simulink model "SimpleBounce"  (Simulink 10.0)
settings: Solver=ode23t  StartTime=0.0  StopTime=3  RelTol=1e-3  EnableMultiTasking=on
libraries: simulink x1, tstbxlib x1
settings Model: Creator=grouleau  LastModifiedBy=bhisma
settings SolverCC: ZeroCrossControl=EnableAll
settings DataIOCC: LimitDataPoints=on  SignalLoggingSaveFormat=ModelDataLogs
settings OptimizationCC: ExpressionDepthLimit=2147483647
settings DebuggingCC: SolverPrmCheckMsg=warning  FcnCallInpInsideContextMsg=warning  StateNameClashWarn=warning
settings GRTTargetCC: GeneratePreprocessorConditionals=Disable all
settings ConfigComp: CovExternalEMLEnable=off

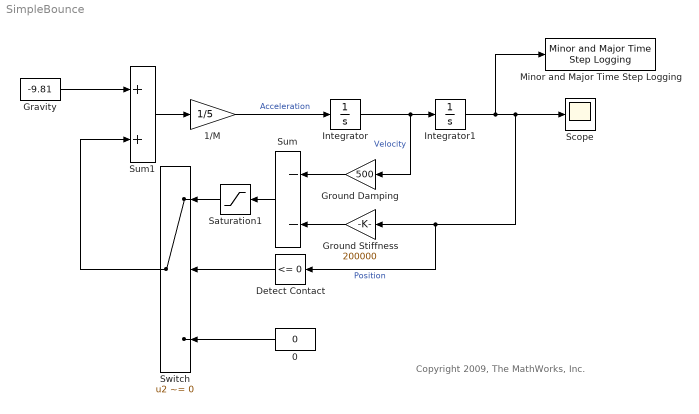
== system SimpleBounce ==
  note: Copyright 2009, The MathWorks, Inc.
  0 : Constant  Value=0
  1/M : Gain  Gain=1/5
  Detect Contact : simulink/Logic and Bit Operations/Compare To Zero  SystemSampleTime=-1  relop=<=  LogicOutDataTypeMode=uint8
  Gravity : Constant  Value=-9.81
  Ground Damping : Gain  Gain=500
  Ground Stiffness : Gain  Gain=200000
  Integrator : Integrator
  Integrator1 : Integrator  InitialCondition=1
  Minor and Major Time Step Logging : tstbxlib/Minor Time Step Logging Library/Minor and Major Time Step Logging  enab=on  minordata=minordata  majordata=majordata  n=999
  Saturation1 : Saturate  UpperLimit=inf  LowerLimit=0
  Scope : Scope
  Sum : Sum  Inputs=--
  Sum1 : Sum
  Switch : Switch  Criteria=u2 ~= 0
  wires:
  1/M/1 -> Integrator/1  "Acceleration"
  Integrator/1 -> Integrator1/1, Ground Damping/1  "Velocity"
  Integrator1/1 -> Scope/1, Ground Stiffness/1, Detect Contact/1, Minor and Major Time Step Logging/1  "Position"
  Ground Damping/1 -> Sum/1
  Ground Stiffness/1 -> Sum/2
  Gravity/1 -> Sum1/1
  Sum1/1 -> 1/M/1
  Detect Contact/1 -> Switch/2
  Sum/1 -> Saturation1/1
  Switch/1 -> Sum1/2
  0/1 -> Switch/3
  Saturation1/1 -> Switch/1
